simulink model "CSWI"  (Simulink 7.8)
settings: Solver=ode3  StartTime=0.0  StopTime=t_sim  FixedStep=1/6400  MaxStep=0.001  MinStep=0.000005  RelTol=1e-3
StopFcn:
  | ComtradeWrite5( RDRE1_UIabc, RDRE1_ANames, RDRE1_Dsignals, RDRE1_DNames, RDRE1_ADCscale, RDRE1_PromtFile, RDRE1_NumFile, RDRE1_FileFormat, RDRE1_TestNum);
  | clear RDRE1_UIabc RDRE1_ANames RDRE1_Dsignals RDRE1_DNames RDRE1_ADCscale  RDRE1_PromtFile RDRE1_NumFile RDRE1_FileFormat RDRE1_TestNum
values from neighbouring files (symbols this model uses):
  BlkTmms1 = 700    [CSWI_SG1.m]    (also in CSWI_SG2.m = 650; CSWI_SG3.m; CSWI_SG4.m; CSWI_SG5.m)
  BlkTmms2 = 800    [CSWI_SG1.m]    (also in CSWI_SG2.m = 750; CSWI_SG3.m; CSWI_SG4.m; CSWI_SG5.m)
  ClsTmms1 = 250    [CSWI_SG1.m]    (also in CSWI_SG2.m = 200; CSWI_SG3.m; CSWI_SG4.m; CSWI_SG5.m)
  ClsTmms2 = 170    [CSWI_SG1.m]    (also in CSWI_SG2.m = 100; CSWI_SG3.m; CSWI_SG4.m; CSWI_SG5.m)
  ClsTmms3 = 60    [CSWI_SG1.m]    (also in CSWI_SG2.m = 30; CSWI_SG3.m; CSWI_SG4.m; CSWI_SG5.m)
  ClsTmms4 = 10    [CSWI_SG1.m]    (also in CSWI_SG2.m = 20; CSWI_SG3.m; CSWI_SG4.m; CSWI_SG5.m)
  FailTmms = 350    [CSWI_SG1.m]    (also in CSWI_SG2.m = 300; CSWI_SG3.m; CSWI_SG4.m; CSWI_SG5.m)
  FctMod1 = 1    [CSWI_SG1.m]    (also in CSWI_SG2.m; CSWI_SG3.m; CSWI_SG4.m; CSWI_SG5.m)
  FctMod2 = 1    [CSWI_SG1.m]    (also in CSWI_SG2.m; CSWI_SG3.m; CSWI_SG4.m = 0; CSWI_SG5.m)
  FctMod3 = 1    [CSWI_SG1.m]    (also in CSWI_SG2.m; CSWI_SG3.m; CSWI_SG4.m; CSWI_SG5.m = 0)
  Num_SG = 1    [CSWI_generate_tests.m]
  OpnTmms1 = 300    [CSWI_SG1.m]    (also in CSWI_SG2.m = 250; CSWI_SG3.m; CSWI_SG4.m; CSWI_SG5.m)
  OpnTmms2 = 200    [CSWI_SG1.m]    (also in CSWI_SG2.m = 150; CSWI_SG3.m; CSWI_SG4.m; CSWI_SG5.m)
  OpnTmms3 = 30    [CSWI_SG1.m]    (also in CSWI_SG2.m = 90; CSWI_SG3.m = 90; CSWI_SG4.m; CSWI_SG5.m)
  test_dc = 'Ïðîâåðêà îòñóòñòâèÿ ôîðìèðîâàíèÿ ñèãíàëîâ "Âêë." ïðè ôîðìèðîâàíèè ñèãíàëà  "Îòêë. îò ÄÓ"'    [CSWI_generate_tests.m]
undefined symbols (not defined in the file or in its folder): sigbuilder_block, Test_num
libraries: powerlib_extras x21
(part 2 of 3)

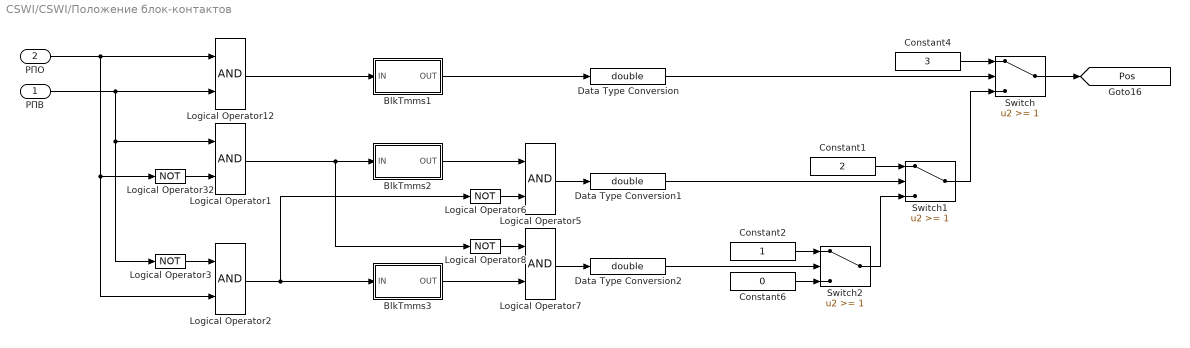
== system CSWI/CSWI/Положение блок-контактов ==
  РПВ : Inport  SampleTime=Tmega
  РПО : Inport  Port=2  SampleTime=Tmega
  BlkTmms1 : Subsystem  DialogController=POWERSYS.PowerSysDialog  mask(Discrete On/Off Delay ){type_delay=On delay, delay=0.5, ic=0, Ts=Tmega}
      mask prompts: type_delay "Type:"; delay "Time delay:"; ic "Input at t = -Ts (0/1):"; Ts "Sample time Ts:"
      mask help:
      | Apply a delay on the input signal when the input changes to TRUE (1) or FALSE (0).
      |
      | On delay: When the input becomes TRUE, the output becomes TRUE after the specified time delay as long as the input is still TRUE. If the input becomes FALSE before the time delay has expired , the output stays FALSE.
      |
      | Off delay: When the input becomes FALSE, the output becomes FALSE after the specified time delay as long as the input is still FALSE. If the input becomes TRUE before the time delay has expired , the output stays TRUE.
      |
      | The input value (0/1) at time step preceding t=0 is specified by the parameter "input at t = -Ts".
      mask init:
      | str=sprintf('%g %c',delay,'s');
      | power_initmask();
      mask Help: This block is part of a subset of blocks in the Extras library that does not have documentation associated with it, other than the block mask description.
      mask StyleString: popup(On delay|Off delay),edit,edit,edit
      mask Display:
      | plot(0,0,100,100,[10,10,10,90,90,90],[60,40,50,50,40,60]);
      | text(25+(type_delay-1)*50,80,'t');
      | text(15,20,str);
  BlkTmms2 : Subsystem  DialogController=POWERSYS.PowerSysDialog  mask(Discrete On/Off Delay ){type_delay=Off delay, delay=0.5, ic=0, Ts=Tmega}
      mask prompts: type_delay "Type:"; delay "Time delay:"; ic "Input at t = -Ts (0/1):"; Ts "Sample time Ts:"
      mask help:
      | Apply a delay on the input signal when the input changes to TRUE (1) or FALSE (0).
      |
      | On delay: When the input becomes TRUE, the output becomes TRUE after the specified time delay as long as the input is still TRUE. If the input becomes FALSE before the time delay has expired , the output stays FALSE.
      |
      | Off delay: When the input becomes FALSE, the output becomes FALSE after the specified time delay as long as the input is still FALSE. If the input becomes TRUE before the time delay has expired , the output stays TRUE.
      |
      | The input value (0/1) at time step preceding t=0 is specified by the parameter "input at t = -Ts".
      mask init:
      | str=sprintf('%g %c',delay,'s');
      | power_initmask();
      mask Help: This block is part of a subset of blocks in the Extras library that does not have documentation associated with it, other than the block mask description.
      mask StyleString: popup(On delay|Off delay),edit,edit,edit
      mask Display:
      | plot(0,0,100,100,[10,10,10,90,90,90],[60,40,50,50,40,60]);
      | text(25+(type_delay-1)*50,80,'t');
      | text(15,20,str);
  BlkTmms3 : Subsystem  DialogController=POWERSYS.PowerSysDialog  mask(Discrete On/Off Delay ){type_delay=Off delay, delay=0.5, ic=0, Ts=Tmega}
      mask prompts: type_delay "Type:"; delay "Time delay:"; ic "Input at t = -Ts (0/1):"; Ts "Sample time Ts:"
      mask help:
      | Apply a delay on the input signal when the input changes to TRUE (1) or FALSE (0).
      |
      | On delay: When the input becomes TRUE, the output becomes TRUE after the specified time delay as long as the input is still TRUE. If the input becomes FALSE before the time delay has expired , the output stays FALSE.
      |
      | Off delay: When the input becomes FALSE, the output becomes FALSE after the specified time delay as long as the input is still FALSE. If the input becomes TRUE before the time delay has expired , the output stays TRUE.
      |
      | The input value (0/1) at time step preceding t=0 is specified by the parameter "input at t = -Ts".
      mask init:
      | str=sprintf('%g %c',delay,'s');
      | power_initmask();
      mask Help: This block is part of a subset of blocks in the Extras library that does not have documentation associated with it, other than the block mask description.
      mask StyleString: popup(On delay|Off delay),edit,edit,edit
      mask Display:
      | plot(0,0,100,100,[10,10,10,90,90,90],[60,40,50,50,40,60]);
      | text(25+(type_delay-1)*50,80,'t');
      | text(15,20,str);
  Constant1 : Constant  Value=2  SampleTime=Tmega
  Constant2 : Constant  SampleTime=Tmega
  Constant4 : Constant  Value=3  SampleTime=Tmega
  Constant6 : Constant  Value=0  SampleTime=Tmega
  Data Type Conversion : DataTypeConversion  OutDataTypeStr=double  SampleTime=Tmega
  Data Type Conversion1 : DataTypeConversion  OutDataTypeStr=double  SampleTime=Tmega
  Data Type Conversion2 : DataTypeConversion  OutDataTypeStr=double  SampleTime=Tmega
  Logical Operator{1..2,5,7,12} (5 alike) : Logic  AllPortsSameDT=off  OutDataTypeStr=boolean  SampleTime=Tmega
  Logical Operator{3,6,8,32} (4 alike) : Logic  Operator=NOT  AllPortsSameDT=off  OutDataTypeStr=boolean  SampleTime=Tmega
  Switch : Switch  Threshold=1  SampleTime=Tmega
  Switch1 : Switch  Threshold=1  SampleTime=Tmega
  Switch2 : Switch  Threshold=1  SampleTime=Tmega
  tag scope: Pos=global
  wires:
  РПО/1 -> Logical Operator12/1, Logical Operator2/2, Logical Operator32/1
  РПВ/1 -> Logical Operator12/2, Logical Operator3/1, Logical Operator1/1
  Logical Operator12/1 -> BlkTmms1/1(IN)
  Logical Operator32/1 -> Logical Operator1/2
  Logical Operator3/1 -> Logical Operator2/1
  Logical Operator1/1 -> BlkTmms2/1(IN), Logical Operator8/1
  Logical Operator2/1 -> BlkTmms3/1(IN), Logical Operator6/1
  BlkTmms2/1(OUT) -> Logical Operator5/1
  Logical Operator6/1 -> Logical Operator5/2
  BlkTmms3/1(OUT) -> Logical Operator7/2
  Logical Operator8/1 -> Logical Operator7/1
  BlkTmms1/1(OUT) -> Data Type Conversion/1
  Constant4/1 -> Switch/1
  Constant1/1 -> Switch1/1
  Logical Operator5/1 -> Data Type Conversion1/1
  Switch1/1 -> Switch/3
  Data Type Conversion/1 -> Switch/2
  Data Type Conversion1/1 -> Switch1/2
  Switch2/1 -> Switch1/3
  Logical Operator7/1 -> Data Type Conversion2/1
  Data Type Conversion2/1 -> Switch2/2
  Constant2/1 -> Switch2/1
  Switch/1 -> [Pos]
  Constant6/1 -> Switch2/3

== system CSWI/CSWI/РФК и Аварийное отключение ==
  Вывод ОУ : Inport  SampleTime=Tmega
  РПВ : Inport  Port=2  SampleTime=Tmega
  РПО : Inport  Port=3  SampleTime=Tmega
  Опер. Откл. : Inport  Port=4  SampleTime=Tmega
  Discrete Bistable7 : Subsystem  DialogController=POWERSYS.PowerSysDialog  mask(Discrete Bistable Flip-Flop (Priority to Set or Reset)){SPSpriority=Reset, ic=0, Ts=Tmega}
      mask prompts: SPSpriority "Priority to input:"; ic "Initial Q output (0/1):"; Ts "Sample time:"
      mask help:
      | SR Flip-Flop block, with priority given either  to the Set  (S) or Reset  (R) input.
      |
      | Priority to Set: If inputs S (set) and R (reset) are TRUE (1) simultaneously, the output Q is set to TRUE (1).
      |
      | Priority to Reset: If inputs S (set) and R (reset) are TRUE (1) simultaneously, the output Q is reset to FALSE (0).
      |
      | The  Q! output  is the complement of the Q output.
      | The initial value of the Q output  is specified by the parameter "Initial Q output".
      mask init:
      | if (SPSpriority==1)   % RESET
      |  str1 = '[R]';
      |  str2 = 'S';
      | else
      | str1= 'R';
      | str2 = '[S]';
      | end
      | power_initmask();
      mask Help: This block is part of a subset of blocks in the Extras library that does not have documentation associated with it, other than the block mask description.
      mask StyleString: popup(Reset|Set),edit,edit
      mask Display:
      | plot(0,0,100,100);
      | text(8,25,str1);
      | text(8,75,str2);
      | text(72,50,'Q');
  Logical Operator29 : Logic  Operator=OR  AllPortsSameDT=off  OutDataTypeStr=boolean  SampleTime=Tmega
  Logical Operator39 : Logic  AllPortsSameDT=off  OutDataTypeStr=boolean  SampleTime=Tmega
  Logical Operator40 : Logic  AllPortsSameDT=off  OutDataTypeStr=boolean  SampleTime=Tmega
  T. Авар. откл. : powerlib_extras/Discrete  Control Blocks/Discrete On//Off Delay  type_delay=On delay  delay=FailTmms  ic=0  Ts=Tmega
  РФК : Outport  SampleTime=Tmega
  Авар. откл. : Outport  Port=2  SampleTime=Tmega
  wires:
  Logical Operator29/1 -> Discrete Bistable7/2(R)
  РПО/1 -> Logical Operator39/2, Logical Operator40/2
  Discrete Bistable7/1(Q) -> Logical Operator40/1, РФК/1
  Logical Operator40/1 -> T. Авар. откл./1
  Вывод ОУ/1 -> Logical Operator39/1
  РПВ/1 -> Discrete Bistable7/1(S)
  T. Авар. откл./1 -> Авар. откл./1
  Logical Operator39/1 -> Logical Operator29/2
  Опер. Откл./1 -> Logical Operator29/1

== system CSWI/DREGOUT1/Signal Builder ==
  Demux : Demux  Tag=STV Demux  Outputs=1
  FromWs : FromWorkspace  Tag=STV FromWs  VariableName=tuvar  SampleTime=0  SigBuilderData=DataTag0  VnvData=DataTag1
      SigBuilderData=|
      | common.afterFinalStr = 'Extrapolate'
      | common.sampleTime = 0
      | dataSet.timeRange = [0 5]
      | dataSet.name = 'Group 1'
      | sbobj.Groups.Name = 'Group 1'
      | sbobj.Groups.Signals.Name = 'Pusk Osc'
      | sbobj.Groups.Signals.XData = [0 0.5 0.5 0.54 0.54 5]
      | sbobj.Groups.Signals.YData = [0 0 1 1 0 0]
      | sbobj.Groups.TimeRange = [0 5]
  Pusk Osc : Outport  Tag=STV Outport
  wires:
  FromWs/1 -> Demux/1
  Demux/1 -> Pusk Osc/1

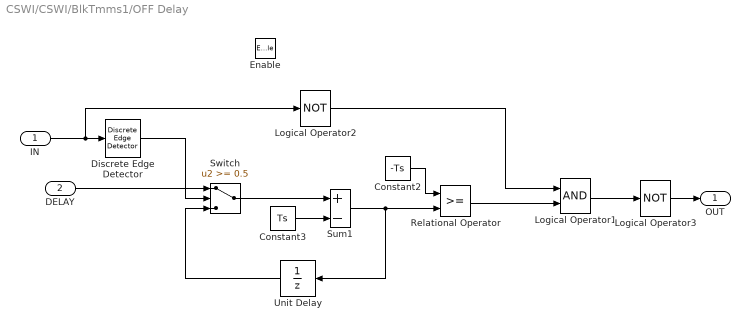
== system CSWI/CSWI/BlkTmms1/OFF Delay ==
  IN : Inport
  DELAY : Inport  Port=2
  Enable : EnablePort  PropagateVarSize=During execution
  Constant2 : Constant  Value=-Ts
  Constant3 : Constant  Value=Ts
  Discrete Edge Detector : powerlib_extras/Discrete  Control Blocks/Discrete Edge Detector  model=Falling  ic=ic  Ts=Ts
  Logical Operator1 : Logic
  Logical Operator2 : Logic  Operator=NOT
  Logical Operator3 : Logic  Operator=NOT
  Relational Operator : RelationalOperator  OutDataTypeStr=boolean  InputSameDT=on
  Sum1 : Sum  Inputs=+-  SaturateOnIntegerOverflow=on  InputSameDT=on  OutDataTypeStr=Inherit: Same as first input
  Switch : Switch  Threshold=0.5  SaturateOnIntegerOverflow=on  InputSameDT=on
  Unit Delay : UnitDelay  SampleTime=Ts
  OUT : Outport
  wires:
  Unit Delay/1 -> Switch/3
  Sum1/1 -> Relational Operator/2, Unit Delay/1
  Switch/1 -> Sum1/1
  Constant3/1 -> Sum1/2
  Relational Operator/1 -> Logical Operator1/2
  IN/1 -> Discrete Edge Detector/1, Logical Operator2/1
  Logical Operator1/1 -> Logical Operator3/1
  DELAY/1 -> Switch/1
  Discrete Edge Detector/1 -> Switch/2
  Constant2/1 -> Relational Operator/1
  Logical Operator2/1 -> Logical Operator1/1
  Logical Operator3/1 -> OUT/1

== system CSWI/CSWI/BlkTmms1/ON Delay ==
  IN : Inport
  DELAY : Inport  Port=2
  Enable : EnablePort  PropagateVarSize=During execution
  Constant2 : Constant  Value=-Ts
  Constant3 : Constant  Value=Ts
  Discrete Edge Detector : powerlib_extras/Discrete  Control Blocks/Discrete Edge Detector  model=Rising  ic=ic  Ts=Ts
  Logical Operator1 : Logic
  Relational Operator : RelationalOperator  OutDataTypeStr=boolean  InputSameDT=on
  Sum1 : Sum  Inputs=+-  SaturateOnIntegerOverflow=on  InputSameDT=on  OutDataTypeStr=Inherit: Same as first input
  Switch : Switch  Threshold=0.5  SaturateOnIntegerOverflow=on  InputSameDT=on
  Unit Delay : UnitDelay  SampleTime=Ts
  OUT : Outport
  wires:
  Unit Delay/1 -> Switch/3
  Sum1/1 -> Unit Delay/1, Relational Operator/2
  Switch/1 -> Sum1/1
  Constant3/1 -> Sum1/2
  Relational Operator/1 -> Logical Operator1/2
  IN/1 -> Discrete Edge Detector/1, Logical Operator1/1
  Logical Operator1/1 -> OUT/1
  DELAY/1 -> Switch/1
  Discrete Edge Detector/1 -> Switch/2
  Constant2/1 -> Relational Operator/1

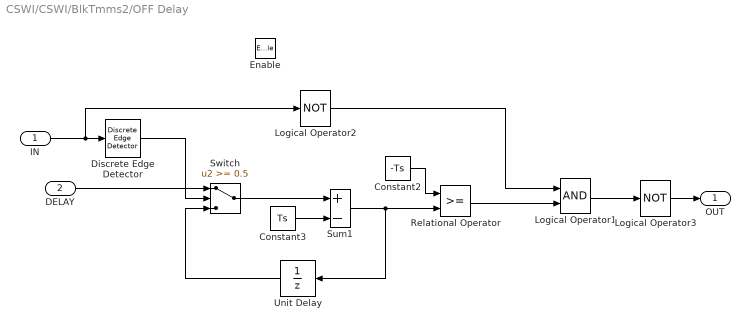
== system CSWI/CSWI/BlkTmms2/OFF Delay ==
  IN : Inport
  DELAY : Inport  Port=2
  Enable : EnablePort  PropagateVarSize=During execution
  Constant2 : Constant  Value=-Ts
  Constant3 : Constant  Value=Ts
  Discrete Edge Detector : powerlib_extras/Discrete  Control Blocks/Discrete Edge Detector  model=Falling  ic=ic  Ts=Ts
  Logical Operator1 : Logic
  Logical Operator2 : Logic  Operator=NOT
  Logical Operator3 : Logic  Operator=NOT
  Relational Operator : RelationalOperator  OutDataTypeStr=boolean  InputSameDT=on
  Sum1 : Sum  Inputs=+-  SaturateOnIntegerOverflow=on  InputSameDT=on  OutDataTypeStr=Inherit: Same as first input
  Switch : Switch  Threshold=0.5  SaturateOnIntegerOverflow=on  InputSameDT=on
  Unit Delay : UnitDelay  SampleTime=Ts
  OUT : Outport
  wires:
  Unit Delay/1 -> Switch/3
  Sum1/1 -> Relational Operator/2, Unit Delay/1
  Switch/1 -> Sum1/1
  Constant3/1 -> Sum1/2
  Relational Operator/1 -> Logical Operator1/2
  IN/1 -> Discrete Edge Detector/1, Logical Operator2/1
  Logical Operator1/1 -> Logical Operator3/1
  DELAY/1 -> Switch/1
  Discrete Edge Detector/1 -> Switch/2
  Constant2/1 -> Relational Operator/1
  Logical Operator2/1 -> Logical Operator1/1
  Logical Operator3/1 -> OUT/1

== system CSWI/CSWI/BlkTmms2/ON Delay ==
  IN : Inport
  DELAY : Inport  Port=2
  Enable : EnablePort  PropagateVarSize=During execution
  Constant2 : Constant  Value=-Ts
  Constant3 : Constant  Value=Ts
  Discrete Edge Detector : powerlib_extras/Discrete  Control Blocks/Discrete Edge Detector  model=Rising  ic=ic  Ts=Ts
  Logical Operator1 : Logic
  Relational Operator : RelationalOperator  OutDataTypeStr=boolean  InputSameDT=on
  Sum1 : Sum  Inputs=+-  SaturateOnIntegerOverflow=on  InputSameDT=on  OutDataTypeStr=Inherit: Same as first input
  Switch : Switch  Threshold=0.5  SaturateOnIntegerOverflow=on  InputSameDT=on
  Unit Delay : UnitDelay  SampleTime=Ts
  OUT : Outport
  wires:
  Unit Delay/1 -> Switch/3
  Sum1/1 -> Unit Delay/1, Relational Operator/2
  Switch/1 -> Sum1/1
  Constant3/1 -> Sum1/2
  Relational Operator/1 -> Logical Operator1/2
  IN/1 -> Discrete Edge Detector/1, Logical Operator1/1
  Logical Operator1/1 -> OUT/1
  DELAY/1 -> Switch/1
  Discrete Edge Detector/1 -> Switch/2
  Constant2/1 -> Relational Operator/1

== system CSWI/CSWI/Блок включения/ClsTmms1 ==
  note: Silvano Casoria
      | Power System Simulation Laboratory
      | IREQ, Hydro-Quebc
  note: Discrete On/Off Delay
  IN : Inport
  Constant : Constant
  Constant1 : Constant  Value=delay - eps
  Constant2 : Constant  Value=type_delay
  Data Type Conversion1 : DataTypeConversion  OutDataTypeStr=boolean  SaturateOnIntegerOverflow=on  RndMeth=Zero
  Logical Operator1 : Logic  Operator=OR
  Logical Operator2 : Logic  Operator=NOT  Inputs=1
  OFF Delay : Subsystem  TreatAsAtomicUnit=on
  ON Delay : Subsystem  TreatAsAtomicUnit=on
  Relational Operator1 : RelationalOperator  Operator===  InputSameDT=on
  OUT : Outport
  wires:
  Data Type Conversion1/1 -> ON Delay/1(IN), OFF Delay/1(IN)
  Constant/1 -> Relational Operator1/2
  Relational Operator1/1 -> ON Delay/Enable, Logical Operator2/1
  Constant2/1 -> Relational Operator1/1
  Logical Operator2/1 -> OFF Delay/Enable
  OFF Delay/1(OUT) -> Logical Operator1/2
  ON Delay/1(OUT) -> Logical Operator1/1
  Logical Operator1/1 -> OUT/1
  Constant1/1 -> ON Delay/2(DELAY), OFF Delay/2(DELAY)
  IN/1 -> Data Type Conversion1/1

== system CSWI/CSWI/Блок включения/ClsTmms2 ==
  note: Discrete Monostable
  note: Silvano Casoria
      | Power System Simulation Laboratory
      | IREQ, Hydro-Quebc
  In : Inport
  Constant2 : Constant  Value=-Ts
  Constant3 : Constant  Value=Ts
  Edge_Detector : Subsystem  mask(Discrete Edge Detector){model=EdgeDetect, ic=ic, Ts=Ts}
      mask prompts: model "Edge:"; ic "Input at t = -Ts:"; Ts "Sample time Ts:"
      mask help:
      | This block compares its present input to its previous input.
      |
      | If the input  is a logic signal (TRUE (1) or FALSE (0), the output is a one-step boolean signal TRUE  when  the specified edge (Rising, Falling or Either)  is detected.
      |
      | This block can also be used to detect the slope polarity of a continuous signal. For example, if the specified edge is  "Rising", the output is TRUE as long as the slope of the input signal is positive.
      |
      | The input value at time step preceding t=0 is specified by the parameter "Input at t=-Ts"
      mask init:
      | if model~=3,
      | 	x1 = (model -1)*20;
      |     x2 = (model -1)*60;
      | 	X1=[5,20,20,35]+25; Y1=[20+x2,20+x2,80-x2,80-x2];
      | 	X2=[5,20,35]+25;    Y2=[40+x1,60-x1,40+x1];
      | 	X3=[];X4=[];Y3=[];Y4=[];
      | else
      | 	x1 = 20;
      | 	x2 = 60;
      | 	X1=[5,20,20,35]+8; Y1=[20,20,80,80];
      | 	X2=[5,20,35]+8;    Y2=[40,60,40];
      | 	X3=[5,20,20,35]+53; Y3=[20+x2,20+x2,80-x2,80-x2];
      | 	X4=[5,20,35]+53;    Y4=[40+x1,60-x1,40+x1];
      | end
      mask Display: plot(0,0,100,100, X1,Y1,X2,Y2,X3,Y3,X4,Y4);
  Logical Operator1 : Logic
  Logical Operator2 : Logic  Operator=NOT  Inputs=1
  Relational Operator : RelationalOperator  Operator=>  InputSameDT=on
  Sum1 : Sum  Inputs=+-  SaturateOnIntegerOverflow=on  InputSameDT=on  OutDataTypeStr=Inherit: Same as first input
  Switch : Switch  Threshold=0.5  SaturateOnIntegerOverflow=on  InputSameDT=on
  T_monostable : Constant  Value=t_mono-eps
  Unit Delay : UnitDelay  SampleTime=Ts
  delay : UnitDelay  SampleTime=Ts
  Out : Outport
  wires:
  Sum1/1 -> Unit Delay/1, Relational Operator/1
  Unit Delay/1 -> Switch/3
  Constant3/1 -> Sum1/2
  Switch/1 -> Sum1/1
  T_monostable/1 -> Switch/1
  In/1 -> Edge_Detector/1(In)
  Relational Operator/1 -> delay/1, Out/1
  Logical Operator1/1 -> Switch/2
  delay/1 -> Logical Operator2/1
  Logical Operator2/1 -> Logical Operator1/1
  Edge_Detector/1(Out) -> Logical Operator1/2
  Constant2/1 -> Relational Operator/2

== system CSWI/CSWI/Блок включения/ClsTmms3 ==
  note: Silvano Casoria
      | Power System Simulation Laboratory
      | IREQ, Hydro-Quebc
  note: Discrete On/Off Delay
  IN : Inport
  Constant : Constant
  Constant1 : Constant  Value=delay - eps
  Constant2 : Constant  Value=type_delay
  Data Type Conversion1 : DataTypeConversion  OutDataTypeStr=boolean  SaturateOnIntegerOverflow=on  RndMeth=Zero
  Logical Operator1 : Logic  Operator=OR
  Logical Operator2 : Logic  Operator=NOT  Inputs=1
  OFF Delay : Subsystem  TreatAsAtomicUnit=on
  ON Delay : Subsystem  TreatAsAtomicUnit=on
  Relational Operator1 : RelationalOperator  Operator===  InputSameDT=on
  OUT : Outport
  wires:
  Data Type Conversion1/1 -> ON Delay/1(IN), OFF Delay/1(IN)
  Constant/1 -> Relational Operator1/2
  Relational Operator1/1 -> ON Delay/Enable, Logical Operator2/1
  Constant2/1 -> Relational Operator1/1
  Logical Operator2/1 -> OFF Delay/Enable
  OFF Delay/1(OUT) -> Logical Operator1/2
  ON Delay/1(OUT) -> Logical Operator1/1
  Logical Operator1/1 -> OUT/1
  Constant1/1 -> ON Delay/2(DELAY), OFF Delay/2(DELAY)
  IN/1 -> Data Type Conversion1/1

== system CSWI/CSWI/Блок включения/ClsTmms4 ==
  note: Silvano Casoria
      | Power System Simulation Laboratory
      | IREQ, Hydro-Quebc
  note: Discrete On/Off Delay
  IN : Inport
  Constant : Constant
  Constant1 : Constant  Value=delay - eps
  Constant2 : Constant  Value=type_delay
  Data Type Conversion1 : DataTypeConversion  OutDataTypeStr=boolean  SaturateOnIntegerOverflow=on  RndMeth=Zero
  Logical Operator1 : Logic  Operator=OR
  Logical Operator2 : Logic  Operator=NOT  Inputs=1
  OFF Delay : Subsystem  TreatAsAtomicUnit=on
  ON Delay : Subsystem  TreatAsAtomicUnit=on
  Relational Operator1 : RelationalOperator  Operator===  InputSameDT=on
  OUT : Outport
  wires:
  Data Type Conversion1/1 -> ON Delay/1(IN), OFF Delay/1(IN)
  Constant/1 -> Relational Operator1/2
  Relational Operator1/1 -> ON Delay/Enable, Logical Operator2/1
  Constant2/1 -> Relational Operator1/1
  Logical Operator2/1 -> OFF Delay/Enable
  OFF Delay/1(OUT) -> Logical Operator1/2
  ON Delay/1(OUT) -> Logical Operator1/1
  Logical Operator1/1 -> OUT/1
  Constant1/1 -> ON Delay/2(DELAY), OFF Delay/2(DELAY)
  IN/1 -> Data Type Conversion1/1

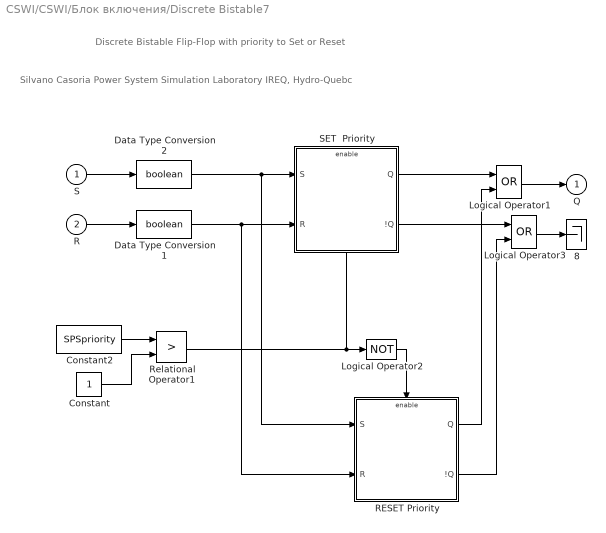
== system CSWI/CSWI/Блок включения/Discrete Bistable7 ==
  note: Silvano Casoria
      | Power System Simulation Laboratory
      | IREQ, Hydro-Quebc
  note: Discrete Bistable Flip-Flop with priority to Set or Reset
  S : Inport
  R : Inport  Port=2
  8 : Terminator
  Constant : Constant
  Constant2 : Constant  Value=SPSpriority
  Data Type Conversion1 : DataTypeConversion  OutDataTypeStr=boolean  SaturateOnIntegerOverflow=on  RndMeth=Zero
  Data Type Conversion2 : DataTypeConversion  OutDataTypeStr=boolean  SaturateOnIntegerOverflow=on  RndMeth=Zero
  Logical Operator1 : Logic  Operator=OR
  Logical Operator2 : Logic  Operator=NOT  Inputs=1
  Logical Operator3 : Logic  Operator=OR
  RESET Priority : Subsystem  TreatAsAtomicUnit=on
  Relational Operator1 : RelationalOperator  Operator=>  InputSameDT=on
  SET  Priority : Subsystem  TreatAsAtomicUnit=on
  Q : Outport  InitialOutput=0
  wires:
  RESET Priority/2(!Q) -> Logical Operator3/2
  RESET Priority/1(Q) -> Logical Operator1/2
  Logical Operator3/1 -> 8/1
  SET  Priority/2(!Q) -> Logical Operator3/1
  Logical Operator1/1 -> Q/1
  SET  Priority/1(Q) -> Logical Operator1/1
  Constant/1 -> Relational Operator1/2
  Relational Operator1/1 -> SET  Priority/Enable, Logical Operator2/1
  Constant2/1 -> Relational Operator1/1
  Logical Operator2/1 -> RESET Priority/Enable
  Data Type Conversion1/1 -> SET  Priority/2(R), RESET Priority/2(R)
  Data Type Conversion2/1 -> SET  Priority/1(S), RESET Priority/1(S)
  S/1 -> Data Type Conversion2/1
  R/1 -> Data Type Conversion1/1

== system CSWI/CSWI/Блок отключения/OpnTmms1 ==
  note: Silvano Casoria
      | Power System Simulation Laboratory
      | IREQ, Hydro-Quebc
  note: Discrete On/Off Delay
  IN : Inport
  Constant : Constant
  Constant1 : Constant  Value=delay - eps
  Constant2 : Constant  Value=type_delay
  Data Type Conversion1 : DataTypeConversion  OutDataTypeStr=boolean  SaturateOnIntegerOverflow=on  RndMeth=Zero
  Logical Operator1 : Logic  Operator=OR
  Logical Operator2 : Logic  Operator=NOT  Inputs=1
  OFF Delay : Subsystem  TreatAsAtomicUnit=on
  ON Delay : Subsystem  TreatAsAtomicUnit=on
  Relational Operator1 : RelationalOperator  Operator===  InputSameDT=on
  OUT : Outport
  wires:
  Data Type Conversion1/1 -> ON Delay/1(IN), OFF Delay/1(IN)
  Constant/1 -> Relational Operator1/2
  Relational Operator1/1 -> ON Delay/Enable, Logical Operator2/1
  Constant2/1 -> Relational Operator1/1
  Logical Operator2/1 -> OFF Delay/Enable
  OFF Delay/1(OUT) -> Logical Operator1/2
  ON Delay/1(OUT) -> Logical Operator1/1
  Logical Operator1/1 -> OUT/1
  Constant1/1 -> ON Delay/2(DELAY), OFF Delay/2(DELAY)
  IN/1 -> Data Type Conversion1/1

== system CSWI/CSWI/Блок отключения/OpnTmms2 ==
  note: Discrete Monostable
  note: Silvano Casoria
      | Power System Simulation Laboratory
      | IREQ, Hydro-Quebc
  In : Inport
  Constant2 : Constant  Value=-Ts
  Constant3 : Constant  Value=Ts
  Edge_Detector : Subsystem  mask(Discrete Edge Detector){model=EdgeDetect, ic=ic, Ts=Ts}
      mask prompts: model "Edge:"; ic "Input at t = -Ts:"; Ts "Sample time Ts:"
      mask help:
      | This block compares its present input to its previous input.
      |
      | If the input  is a logic signal (TRUE (1) or FALSE (0), the output is a one-step boolean signal TRUE  when  the specified edge (Rising, Falling or Either)  is detected.
      |
      | This block can also be used to detect the slope polarity of a continuous signal. For example, if the specified edge is  "Rising", the output is TRUE as long as the slope of the input signal is positive.
      |
      | The input value at time step preceding t=0 is specified by the parameter "Input at t=-Ts"
      mask init: same as CSWI/CSWI/Блок включения/ClsTmms2/Edge_Detector
      mask Display: plot(0,0,100,100, X1,Y1,X2,Y2,X3,Y3,X4,Y4);
  Logical Operator1 : Logic
  Logical Operator2 : Logic  Operator=NOT  Inputs=1
  Relational Operator : RelationalOperator  Operator=>  InputSameDT=on
  Sum1 : Sum  Inputs=+-  SaturateOnIntegerOverflow=on  InputSameDT=on  OutDataTypeStr=Inherit: Same as first input
  Switch : Switch  Threshold=0.5  SaturateOnIntegerOverflow=on  InputSameDT=on
  T_monostable : Constant  Value=t_mono-eps
  Unit Delay : UnitDelay  SampleTime=Ts
  delay : UnitDelay  SampleTime=Ts
  Out : Outport
  wires:
  Sum1/1 -> Unit Delay/1, Relational Operator/1
  Unit Delay/1 -> Switch/3
  Constant3/1 -> Sum1/2
  Switch/1 -> Sum1/1
  T_monostable/1 -> Switch/1
  In/1 -> Edge_Detector/1(In)
  Relational Operator/1 -> delay/1, Out/1
  Logical Operator1/1 -> Switch/2
  delay/1 -> Logical Operator2/1
  Logical Operator2/1 -> Logical Operator1/1
  Edge_Detector/1(Out) -> Logical Operator1/2
  Constant2/1 -> Relational Operator/2

== system CSWI/CSWI/Блок отключения/OpnTmms3 ==
  note: Silvano Casoria
      | Power System Simulation Laboratory
      | IREQ, Hydro-Quebc
  note: Discrete On/Off Delay
  IN : Inport
  Constant : Constant
  Constant1 : Constant  Value=delay - eps
  Constant2 : Constant  Value=type_delay
  Data Type Conversion1 : DataTypeConversion  OutDataTypeStr=boolean  SaturateOnIntegerOverflow=on  RndMeth=Zero
  Logical Operator1 : Logic  Operator=OR
  Logical Operator2 : Logic  Operator=NOT  Inputs=1
  OFF Delay : Subsystem  TreatAsAtomicUnit=on
  ON Delay : Subsystem  TreatAsAtomicUnit=on
  Relational Operator1 : RelationalOperator  Operator===  InputSameDT=on
  OUT : Outport
  wires:
  Data Type Conversion1/1 -> ON Delay/1(IN), OFF Delay/1(IN)
  Constant/1 -> Relational Operator1/2
  Relational Operator1/1 -> ON Delay/Enable, Logical Operator2/1
  Constant2/1 -> Relational Operator1/1
  Logical Operator2/1 -> OFF Delay/Enable
  OFF Delay/1(OUT) -> Logical Operator1/2
  ON Delay/1(OUT) -> Logical Operator1/1
  Logical Operator1/1 -> OUT/1
  Constant1/1 -> ON Delay/2(DELAY), OFF Delay/2(DELAY)
  IN/1 -> Data Type Conversion1/1

== system CSWI/CSWI/Положение блок-контактов/BlkTmms1 ==
  note: Silvano Casoria
      | Power System Simulation Laboratory
      | IREQ, Hydro-Quebc
  note: Discrete On/Off Delay
  IN : Inport  SampleTime=Tmega
  Constant : Constant  SampleTime=Tmega
  Constant1 : Constant  Value=delay - eps  SampleTime=Tmega
  Constant2 : Constant  Value=type_delay  SampleTime=Tmega
  Data Type Conversion1 : DataTypeConversion  OutDataTypeStr=boolean  SampleTime=Tmega  SaturateOnIntegerOverflow=on  RndMeth=Zero
  Logical Operator1 : Logic  Operator=OR  SampleTime=Tmega
  Logical Operator2 : Logic  Operator=NOT  Inputs=1  SampleTime=Tmega
  OFF Delay : Subsystem  TreatAsAtomicUnit=on
  ON Delay : Subsystem  TreatAsAtomicUnit=on
  Relational Operator1 : RelationalOperator  Operator===  SampleTime=Tmega  InputSameDT=on
  OUT : Outport  SampleTime=Tmega
  wires:
  Data Type Conversion1/1 -> ON Delay/1(IN), OFF Delay/1(IN)
  Constant/1 -> Relational Operator1/2
  Relational Operator1/1 -> ON Delay/Enable, Logical Operator2/1
  Constant2/1 -> Relational Operator1/1
  Logical Operator2/1 -> OFF Delay/Enable
  OFF Delay/1(OUT) -> Logical Operator1/2
  ON Delay/1(OUT) -> Logical Operator1/1
  Logical Operator1/1 -> OUT/1
  Constant1/1 -> ON Delay/2(DELAY), OFF Delay/2(DELAY)
  IN/1 -> Data Type Conversion1/1

== system CSWI/CSWI/Положение блок-контактов/BlkTmms2 ==
  note: Silvano Casoria
      | Power System Simulation Laboratory
      | IREQ, Hydro-Quebc
  note: Discrete On/Off Delay
  IN : Inport  SampleTime=Tmega
  Constant : Constant  SampleTime=Tmega
  Constant1 : Constant  Value=delay - eps  SampleTime=Tmega
  Constant2 : Constant  Value=type_delay  SampleTime=Tmega
  Data Type Conversion1 : DataTypeConversion  OutDataTypeStr=boolean  SampleTime=Tmega  SaturateOnIntegerOverflow=on  RndMeth=Zero
  Logical Operator1 : Logic  Operator=OR  SampleTime=Tmega
  Logical Operator2 : Logic  Operator=NOT  Inputs=1  SampleTime=Tmega
  OFF Delay : Subsystem  TreatAsAtomicUnit=on
  ON Delay : Subsystem  TreatAsAtomicUnit=on
  Relational Operator1 : RelationalOperator  Operator===  SampleTime=Tmega  InputSameDT=on
  OUT : Outport  SampleTime=Tmega
  wires:
  Data Type Conversion1/1 -> ON Delay/1(IN), OFF Delay/1(IN)
  Constant/1 -> Relational Operator1/2
  Relational Operator1/1 -> ON Delay/Enable, Logical Operator2/1
  Constant2/1 -> Relational Operator1/1
  Logical Operator2/1 -> OFF Delay/Enable
  OFF Delay/1(OUT) -> Logical Operator1/2
  ON Delay/1(OUT) -> Logical Operator1/1
  Logical Operator1/1 -> OUT/1
  Constant1/1 -> ON Delay/2(DELAY), OFF Delay/2(DELAY)
  IN/1 -> Data Type Conversion1/1

== system CSWI/CSWI/Положение блок-контактов/BlkTmms3 ==
  note: Silvano Casoria
      | Power System Simulation Laboratory
      | IREQ, Hydro-Quebc
  note: Discrete On/Off Delay
  IN : Inport  SampleTime=Tmega
  Constant : Constant  SampleTime=Tmega
  Constant1 : Constant  Value=delay - eps  SampleTime=Tmega
  Constant2 : Constant  Value=type_delay  SampleTime=Tmega
  Data Type Conversion1 : DataTypeConversion  OutDataTypeStr=boolean  SampleTime=Tmega  SaturateOnIntegerOverflow=on  RndMeth=Zero
  Logical Operator1 : Logic  Operator=OR  SampleTime=Tmega
  Logical Operator2 : Logic  Operator=NOT  Inputs=1  SampleTime=Tmega
  OFF Delay : Subsystem  TreatAsAtomicUnit=on
  ON Delay : Subsystem  TreatAsAtomicUnit=on
  Relational Operator1 : RelationalOperator  Operator===  SampleTime=Tmega  InputSameDT=on
  OUT : Outport  SampleTime=Tmega
  wires:
  Data Type Conversion1/1 -> ON Delay/1(IN), OFF Delay/1(IN)
  Constant/1 -> Relational Operator1/2
  Relational Operator1/1 -> ON Delay/Enable, Logical Operator2/1
  Constant2/1 -> Relational Operator1/1
  Logical Operator2/1 -> OFF Delay/Enable
  OFF Delay/1(OUT) -> Logical Operator1/2
  ON Delay/1(OUT) -> Logical Operator1/1
  Logical Operator1/1 -> OUT/1
  Constant1/1 -> ON Delay/2(DELAY), OFF Delay/2(DELAY)
  IN/1 -> Data Type Conversion1/1

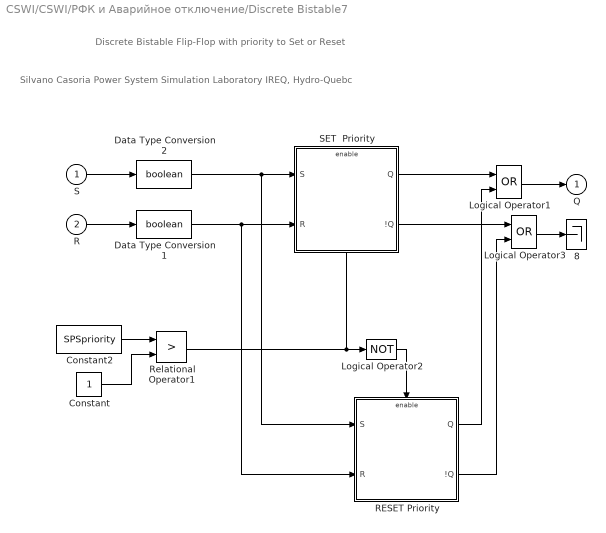
== system CSWI/CSWI/РФК и Аварийное отключение/Discrete Bistable7 ==
  note: Silvano Casoria
      | Power System Simulation Laboratory
      | IREQ, Hydro-Quebc
  note: Discrete Bistable Flip-Flop with priority to Set or Reset
  S : Inport
  R : Inport  Port=2
  8 : Terminator
  Constant : Constant
  Constant2 : Constant  Value=SPSpriority
  Data Type Conversion1 : DataTypeConversion  OutDataTypeStr=boolean  SaturateOnIntegerOverflow=on  RndMeth=Zero
  Data Type Conversion2 : DataTypeConversion  OutDataTypeStr=boolean  SaturateOnIntegerOverflow=on  RndMeth=Zero
  Logical Operator1 : Logic  Operator=OR
  Logical Operator2 : Logic  Operator=NOT  Inputs=1
  Logical Operator3 : Logic  Operator=OR
  RESET Priority : Subsystem  TreatAsAtomicUnit=on
  Relational Operator1 : RelationalOperator  Operator=>  InputSameDT=on
  SET  Priority : Subsystem  TreatAsAtomicUnit=on
  Q : Outport  InitialOutput=0
  wires:
  RESET Priority/2(!Q) -> Logical Operator3/2
  RESET Priority/1(Q) -> Logical Operator1/2
  Logical Operator3/1 -> 8/1
  SET  Priority/2(!Q) -> Logical Operator3/1
  Logical Operator1/1 -> Q/1
  SET  Priority/1(Q) -> Logical Operator1/1
  Constant/1 -> Relational Operator1/2
  Relational Operator1/1 -> SET  Priority/Enable, Logical Operator2/1
  Constant2/1 -> Relational Operator1/1
  Logical Operator2/1 -> RESET Priority/Enable
  Data Type Conversion1/1 -> SET  Priority/2(R), RESET Priority/2(R)
  Data Type Conversion2/1 -> SET  Priority/1(S), RESET Priority/1(S)
  S/1 -> Data Type Conversion2/1
  R/1 -> Data Type Conversion1/1

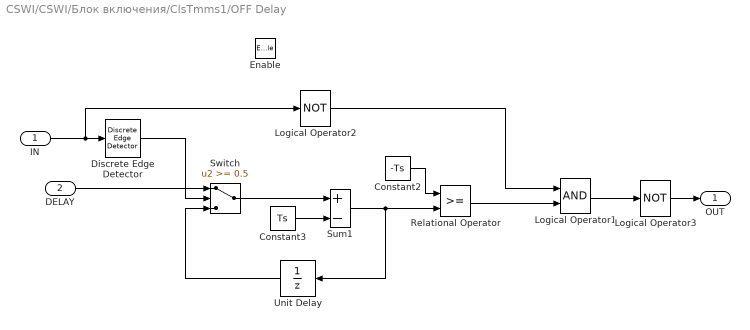
== system CSWI/CSWI/Блок включения/ClsTmms1/OFF Delay ==
  IN : Inport
  DELAY : Inport  Port=2
  Enable : EnablePort  PropagateVarSize=During execution
  Constant2 : Constant  Value=-Ts
  Constant3 : Constant  Value=Ts
  Discrete Edge Detector : powerlib_extras/Discrete  Control Blocks/Discrete Edge Detector  model=Falling  ic=ic  Ts=Ts
  Logical Operator1 : Logic
  Logical Operator2 : Logic  Operator=NOT
  Logical Operator3 : Logic  Operator=NOT
  Relational Operator : RelationalOperator  OutDataTypeStr=boolean  InputSameDT=on
  Sum1 : Sum  Inputs=+-  SaturateOnIntegerOverflow=on  InputSameDT=on  OutDataTypeStr=Inherit: Same as first input
  Switch : Switch  Threshold=0.5  SaturateOnIntegerOverflow=on  InputSameDT=on
  Unit Delay : UnitDelay  SampleTime=Ts
  OUT : Outport
  wires:
  Unit Delay/1 -> Switch/3
  Sum1/1 -> Relational Operator/2, Unit Delay/1
  Switch/1 -> Sum1/1
  Constant3/1 -> Sum1/2
  Relational Operator/1 -> Logical Operator1/2
  IN/1 -> Discrete Edge Detector/1, Logical Operator2/1
  Logical Operator1/1 -> Logical Operator3/1
  DELAY/1 -> Switch/1
  Discrete Edge Detector/1 -> Switch/2
  Constant2/1 -> Relational Operator/1
  Logical Operator2/1 -> Logical Operator1/1
  Logical Operator3/1 -> OUT/1

== system CSWI/CSWI/Блок включения/ClsTmms1/ON Delay ==
  IN : Inport
  DELAY : Inport  Port=2
  Enable : EnablePort  PropagateVarSize=During execution
  Constant2 : Constant  Value=-Ts
  Constant3 : Constant  Value=Ts
  Discrete Edge Detector : powerlib_extras/Discrete  Control Blocks/Discrete Edge Detector  model=Rising  ic=ic  Ts=Ts
  Logical Operator1 : Logic
  Relational Operator : RelationalOperator  OutDataTypeStr=boolean  InputSameDT=on
  Sum1 : Sum  Inputs=+-  SaturateOnIntegerOverflow=on  InputSameDT=on  OutDataTypeStr=Inherit: Same as first input
  Switch : Switch  Threshold=0.5  SaturateOnIntegerOverflow=on  InputSameDT=on
  Unit Delay : UnitDelay  SampleTime=Ts
  OUT : Outport
  wires:
  Unit Delay/1 -> Switch/3
  Sum1/1 -> Unit Delay/1, Relational Operator/2
  Switch/1 -> Sum1/1
  Constant3/1 -> Sum1/2
  Relational Operator/1 -> Logical Operator1/2
  IN/1 -> Discrete Edge Detector/1, Logical Operator1/1
  Logical Operator1/1 -> OUT/1
  DELAY/1 -> Switch/1
  Discrete Edge Detector/1 -> Switch/2
  Constant2/1 -> Relational Operator/1

== system CSWI/CSWI/Блок включения/ClsTmms2/Edge_Detector ==
  note: Edge or Slope Detector
  note: Silvano Casoria
      | Power System Simulation Laboratory
      | IREQ, Hydro-Quebc
  In : Inport
  Constant1 : Constant  Value=model
  Demux : Demux  Outputs=2
  Logical Operator1 : Logic  Operator=OR
  Multiport Switch : MultiPortSwitch  zeroidx=off  SaturateOnIntegerOverflow=on
  NEGATIVE Edge : Subsystem  AncestorBlock=extra_sc/Edge/POSITIVE Edge  TreatAsAtomicUnit=on
  POSITIVE Edge : Subsystem  AncestorBlock=extra_sc/Delay_discrete/OFF Delay  TreatAsAtomicUnit=on
  Unit Delay : UnitDelay  X0=ic  SampleTime=Ts
  either edge : Constant  Value=[1 1]
  neg. edge : Constant  Value=[0 1]
  pos. edge : Constant  Value=[1 0]
  Out : Outport
  wires:
  either edge/1 -> Multiport Switch/4
  Demux/2 -> NEGATIVE Edge/Enable
  Demux/1 -> POSITIVE Edge/Enable
  Multiport Switch/1 -> Demux/1
  Constant1/1 -> Multiport Switch/1
  neg. edge/1 -> Multiport Switch/3
  pos. edge/1 -> Multiport Switch/2
  In/1 -> Unit Delay/1, NEGATIVE Edge/1(IN), POSITIVE Edge/1(IN)
  Unit Delay/1 -> NEGATIVE Edge/2(IN previous), POSITIVE Edge/2(IN previous)
  POSITIVE Edge/1(OUT) -> Logical Operator1/1
  NEGATIVE Edge/1(OUT) -> Logical Operator1/2
  Logical Operator1/1 -> Out/1

== system CSWI/CSWI/Блок включения/ClsTmms3/OFF Delay ==
  IN : Inport
  DELAY : Inport  Port=2
  Enable : EnablePort  PropagateVarSize=During execution
  Constant2 : Constant  Value=-Ts
  Constant3 : Constant  Value=Ts
  Discrete Edge Detector : powerlib_extras/Discrete  Control Blocks/Discrete Edge Detector  model=Falling  ic=ic  Ts=Ts
  Logical Operator1 : Logic
  Logical Operator2 : Logic  Operator=NOT
  Logical Operator3 : Logic  Operator=NOT
  Relational Operator : RelationalOperator  OutDataTypeStr=boolean  InputSameDT=on
  Sum1 : Sum  Inputs=+-  SaturateOnIntegerOverflow=on  InputSameDT=on  OutDataTypeStr=Inherit: Same as first input
  Switch : Switch  Threshold=0.5  SaturateOnIntegerOverflow=on  InputSameDT=on
  Unit Delay : UnitDelay  SampleTime=Ts
  OUT : Outport
  wires:
  Unit Delay/1 -> Switch/3
  Sum1/1 -> Relational Operator/2, Unit Delay/1
  Switch/1 -> Sum1/1
  Constant3/1 -> Sum1/2
  Relational Operator/1 -> Logical Operator1/2
  IN/1 -> Discrete Edge Detector/1, Logical Operator2/1
  Logical Operator1/1 -> Logical Operator3/1
  DELAY/1 -> Switch/1
  Discrete Edge Detector/1 -> Switch/2
  Constant2/1 -> Relational Operator/1
  Logical Operator2/1 -> Logical Operator1/1
  Logical Operator3/1 -> OUT/1

== system CSWI/CSWI/Блок включения/ClsTmms3/ON Delay ==
  IN : Inport
  DELAY : Inport  Port=2
  Enable : EnablePort  PropagateVarSize=During execution
  Constant2 : Constant  Value=-Ts
  Constant3 : Constant  Value=Ts
  Discrete Edge Detector : powerlib_extras/Discrete  Control Blocks/Discrete Edge Detector  model=Rising  ic=ic  Ts=Ts
  Logical Operator1 : Logic
  Relational Operator : RelationalOperator  OutDataTypeStr=boolean  InputSameDT=on
  Sum1 : Sum  Inputs=+-  SaturateOnIntegerOverflow=on  InputSameDT=on  OutDataTypeStr=Inherit: Same as first input
  Switch : Switch  Threshold=0.5  SaturateOnIntegerOverflow=on  InputSameDT=on
  Unit Delay : UnitDelay  SampleTime=Ts
  OUT : Outport
  wires:
  Unit Delay/1 -> Switch/3
  Sum1/1 -> Unit Delay/1, Relational Operator/2
  Switch/1 -> Sum1/1
  Constant3/1 -> Sum1/2
  Relational Operator/1 -> Logical Operator1/2
  IN/1 -> Discrete Edge Detector/1, Logical Operator1/1
  Logical Operator1/1 -> OUT/1
  DELAY/1 -> Switch/1
  Discrete Edge Detector/1 -> Switch/2
  Constant2/1 -> Relational Operator/1

== system CSWI/CSWI/Блок включения/ClsTmms4/OFF Delay ==
  IN : Inport
  DELAY : Inport  Port=2
  Enable : EnablePort  PropagateVarSize=During execution
  Constant2 : Constant  Value=-Ts
  Constant3 : Constant  Value=Ts
  Discrete Edge Detector : powerlib_extras/Discrete  Control Blocks/Discrete Edge Detector  model=Falling  ic=ic  Ts=Ts
  Logical Operator1 : Logic
  Logical Operator2 : Logic  Operator=NOT
  Logical Operator3 : Logic  Operator=NOT
  Relational Operator : RelationalOperator  OutDataTypeStr=boolean  InputSameDT=on
  Sum1 : Sum  Inputs=+-  SaturateOnIntegerOverflow=on  InputSameDT=on  OutDataTypeStr=Inherit: Same as first input
  Switch : Switch  Threshold=0.5  SaturateOnIntegerOverflow=on  InputSameDT=on
  Unit Delay : UnitDelay  SampleTime=Ts
  OUT : Outport
  wires:
  Unit Delay/1 -> Switch/3
  Sum1/1 -> Relational Operator/2, Unit Delay/1
  Switch/1 -> Sum1/1
  Constant3/1 -> Sum1/2
  Relational Operator/1 -> Logical Operator1/2
  IN/1 -> Discrete Edge Detector/1, Logical Operator2/1
  Logical Operator1/1 -> Logical Operator3/1
  DELAY/1 -> Switch/1
  Discrete Edge Detector/1 -> Switch/2
  Constant2/1 -> Relational Operator/1
  Logical Operator2/1 -> Logical Operator1/1
  Logical Operator3/1 -> OUT/1

== system CSWI/CSWI/Блок включения/ClsTmms4/ON Delay ==
  IN : Inport
  DELAY : Inport  Port=2
  Enable : EnablePort  PropagateVarSize=During execution
  Constant2 : Constant  Value=-Ts
  Constant3 : Constant  Value=Ts
  Discrete Edge Detector : powerlib_extras/Discrete  Control Blocks/Discrete Edge Detector  model=Rising  ic=ic  Ts=Ts
  Logical Operator1 : Logic
  Relational Operator : RelationalOperator  OutDataTypeStr=boolean  InputSameDT=on
  Sum1 : Sum  Inputs=+-  SaturateOnIntegerOverflow=on  InputSameDT=on  OutDataTypeStr=Inherit: Same as first input
  Switch : Switch  Threshold=0.5  SaturateOnIntegerOverflow=on  InputSameDT=on
  Unit Delay : UnitDelay  SampleTime=Ts
  OUT : Outport
  wires:
  Unit Delay/1 -> Switch/3
  Sum1/1 -> Unit Delay/1, Relational Operator/2
  Switch/1 -> Sum1/1
  Constant3/1 -> Sum1/2
  Relational Operator/1 -> Logical Operator1/2
  IN/1 -> Discrete Edge Detector/1, Logical Operator1/1
  Logical Operator1/1 -> OUT/1
  DELAY/1 -> Switch/1
  Discrete Edge Detector/1 -> Switch/2
  Constant2/1 -> Relational Operator/1

== system CSWI/CSWI/Блок включения/Discrete Bistable7/RESET Priority ==
  S : Inport
  R : Inport  Port=2
  Enable : EnablePort  PropagateVarSize=During execution
  IC = ic : UnitDelay  X0=ic  SampleTime=Ts
  Logical Operator : Logic  Operator=OR
  Logical Operator1 : Logic  Operator=NOT  Inputs=1
  Logical Operator2 : Logic
  Logical Operator3 : Logic  Operator=NOT  Inputs=1
  Q : Outport
  !Q : Outport  Port=2
  wires:
  Logical Operator2/1 -> Q/1, Logical Operator3/1, IC = ic/1
  Logical Operator1/1 -> Logical Operator2/2
  R/1 -> Logical Operator1/1
  Logical Operator/1 -> Logical Operator2/1
  IC = ic/1 -> Logical Operator/2
  Logical Operator3/1 -> !Q/1
  S/1 -> Logical Operator/1

== system CSWI/CSWI/Блок включения/Discrete Bistable7/SET  Priority ==
  S : Inport
  R : Inport  Port=2
  Enable : EnablePort  PropagateVarSize=During execution
  IC = ic : UnitDelay  X0=ic  SampleTime=Ts
  Logical Operator : Logic  Operator=OR
  Logical Operator1 : Logic  Operator=NOT  Inputs=1
  Logical Operator2 : Logic
  Logical Operator3 : Logic  Operator=NOT  Inputs=1
  Q : Outport
  !Q : Outport  Port=2
  wires:
  S/1 -> Logical Operator/1
  Logical Operator3/1 -> !Q/1
  Logical Operator/1 -> IC = ic/1, Logical Operator3/1, Q/1
  R/1 -> Logical Operator1/1
  Logical Operator1/1 -> Logical Operator2/1
  IC = ic/1 -> Logical Operator2/2
  Logical Operator2/1 -> Logical Operator/2

== system CSWI/CSWI/Блок отключения/OpnTmms1/OFF Delay ==
  IN : Inport
  DELAY : Inport  Port=2
  Enable : EnablePort  PropagateVarSize=During execution
  Constant2 : Constant  Value=-Ts
  Constant3 : Constant  Value=Ts
  Discrete Edge Detector : powerlib_extras/Discrete  Control Blocks/Discrete Edge Detector  model=Falling  ic=ic  Ts=Ts
  Logical Operator1 : Logic
  Logical Operator2 : Logic  Operator=NOT
  Logical Operator3 : Logic  Operator=NOT
  Relational Operator : RelationalOperator  OutDataTypeStr=boolean  InputSameDT=on
  Sum1 : Sum  Inputs=+-  SaturateOnIntegerOverflow=on  InputSameDT=on  OutDataTypeStr=Inherit: Same as first input
  Switch : Switch  Threshold=0.5  SaturateOnIntegerOverflow=on  InputSameDT=on
  Unit Delay : UnitDelay  SampleTime=Ts
  OUT : Outport
  wires:
  Unit Delay/1 -> Switch/3
  Sum1/1 -> Relational Operator/2, Unit Delay/1
  Switch/1 -> Sum1/1
  Constant3/1 -> Sum1/2
  Relational Operator/1 -> Logical Operator1/2
  IN/1 -> Discrete Edge Detector/1, Logical Operator2/1
  Logical Operator1/1 -> Logical Operator3/1
  DELAY/1 -> Switch/1
  Discrete Edge Detector/1 -> Switch/2
  Constant2/1 -> Relational Operator/1
  Logical Operator2/1 -> Logical Operator1/1
  Logical Operator3/1 -> OUT/1

== system CSWI/CSWI/Блок отключения/OpnTmms1/ON Delay ==
  IN : Inport
  DELAY : Inport  Port=2
  Enable : EnablePort  PropagateVarSize=During execution
  Constant2 : Constant  Value=-Ts
  Constant3 : Constant  Value=Ts
  Discrete Edge Detector : powerlib_extras/Discrete  Control Blocks/Discrete Edge Detector  model=Rising  ic=ic  Ts=Ts
  Logical Operator1 : Logic
  Relational Operator : RelationalOperator  OutDataTypeStr=boolean  InputSameDT=on
  Sum1 : Sum  Inputs=+-  SaturateOnIntegerOverflow=on  InputSameDT=on  OutDataTypeStr=Inherit: Same as first input
  Switch : Switch  Threshold=0.5  SaturateOnIntegerOverflow=on  InputSameDT=on
  Unit Delay : UnitDelay  SampleTime=Ts
  OUT : Outport
  wires:
  Unit Delay/1 -> Switch/3
  Sum1/1 -> Unit Delay/1, Relational Operator/2
  Switch/1 -> Sum1/1
  Constant3/1 -> Sum1/2
  Relational Operator/1 -> Logical Operator1/2
  IN/1 -> Discrete Edge Detector/1, Logical Operator1/1
  Logical Operator1/1 -> OUT/1
  DELAY/1 -> Switch/1
  Discrete Edge Detector/1 -> Switch/2
  Constant2/1 -> Relational Operator/1

== system CSWI/CSWI/Блок отключения/OpnTmms2/Edge_Detector ==
  note: Edge or Slope Detector
  note: Silvano Casoria
      | Power System Simulation Laboratory
      | IREQ, Hydro-Quebc
  In : Inport
  Constant1 : Constant  Value=model
  Demux : Demux  Outputs=2
  Logical Operator1 : Logic  Operator=OR
  Multiport Switch : MultiPortSwitch  zeroidx=off  SaturateOnIntegerOverflow=on
  NEGATIVE Edge : Subsystem  AncestorBlock=extra_sc/Edge/POSITIVE Edge  TreatAsAtomicUnit=on
  POSITIVE Edge : Subsystem  AncestorBlock=extra_sc/Delay_discrete/OFF Delay  TreatAsAtomicUnit=on
  Unit Delay : UnitDelay  X0=ic  SampleTime=Ts
  either edge : Constant  Value=[1 1]
  neg. edge : Constant  Value=[0 1]
  pos. edge : Constant  Value=[1 0]
  Out : Outport
  wires:
  either edge/1 -> Multiport Switch/4
  Demux/2 -> NEGATIVE Edge/Enable
  Demux/1 -> POSITIVE Edge/Enable
  Multiport Switch/1 -> Demux/1
  Constant1/1 -> Multiport Switch/1
  neg. edge/1 -> Multiport Switch/3
  pos. edge/1 -> Multiport Switch/2
  In/1 -> Unit Delay/1, NEGATIVE Edge/1(IN), POSITIVE Edge/1(IN)
  Unit Delay/1 -> NEGATIVE Edge/2(IN previous), POSITIVE Edge/2(IN previous)
  POSITIVE Edge/1(OUT) -> Logical Operator1/1
  NEGATIVE Edge/1(OUT) -> Logical Operator1/2
  Logical Operator1/1 -> Out/1

== system CSWI/CSWI/Блок отключения/OpnTmms3/OFF Delay ==
  IN : Inport
  DELAY : Inport  Port=2
  Enable : EnablePort  PropagateVarSize=During execution
  Constant2 : Constant  Value=-Ts
  Constant3 : Constant  Value=Ts
  Discrete Edge Detector : powerlib_extras/Discrete  Control Blocks/Discrete Edge Detector  model=Falling  ic=ic  Ts=Ts
  Logical Operator1 : Logic
  Logical Operator2 : Logic  Operator=NOT
  Logical Operator3 : Logic  Operator=NOT
  Relational Operator : RelationalOperator  OutDataTypeStr=boolean  InputSameDT=on
  Sum1 : Sum  Inputs=+-  SaturateOnIntegerOverflow=on  InputSameDT=on  OutDataTypeStr=Inherit: Same as first input
  Switch : Switch  Threshold=0.5  SaturateOnIntegerOverflow=on  InputSameDT=on
  Unit Delay : UnitDelay  SampleTime=Ts
  OUT : Outport
  wires:
  Unit Delay/1 -> Switch/3
  Sum1/1 -> Relational Operator/2, Unit Delay/1
  Switch/1 -> Sum1/1
  Constant3/1 -> Sum1/2
  Relational Operator/1 -> Logical Operator1/2
  IN/1 -> Discrete Edge Detector/1, Logical Operator2/1
  Logical Operator1/1 -> Logical Operator3/1
  DELAY/1 -> Switch/1
  Discrete Edge Detector/1 -> Switch/2
  Constant2/1 -> Relational Operator/1
  Logical Operator2/1 -> Logical Operator1/1
  Logical Operator3/1 -> OUT/1

== system CSWI/CSWI/Блок отключения/OpnTmms3/ON Delay ==
  IN : Inport
  DELAY : Inport  Port=2
  Enable : EnablePort  PropagateVarSize=During execution
  Constant2 : Constant  Value=-Ts
  Constant3 : Constant  Value=Ts
  Discrete Edge Detector : powerlib_extras/Discrete  Control Blocks/Discrete Edge Detector  model=Rising  ic=ic  Ts=Ts
  Logical Operator1 : Logic
  Relational Operator : RelationalOperator  OutDataTypeStr=boolean  InputSameDT=on
  Sum1 : Sum  Inputs=+-  SaturateOnIntegerOverflow=on  InputSameDT=on  OutDataTypeStr=Inherit: Same as first input
  Switch : Switch  Threshold=0.5  SaturateOnIntegerOverflow=on  InputSameDT=on
  Unit Delay : UnitDelay  SampleTime=Ts
  OUT : Outport
  wires:
  Unit Delay/1 -> Switch/3
  Sum1/1 -> Unit Delay/1, Relational Operator/2
  Switch/1 -> Sum1/1
  Constant3/1 -> Sum1/2
  Relational Operator/1 -> Logical Operator1/2
  IN/1 -> Discrete Edge Detector/1, Logical Operator1/1
  Logical Operator1/1 -> OUT/1
  DELAY/1 -> Switch/1
  Discrete Edge Detector/1 -> Switch/2
  Constant2/1 -> Relational Operator/1

== system CSWI/CSWI/Положение блок-контактов/BlkTmms1/OFF Delay ==
  IN : Inport
  DELAY : Inport  Port=2
  Enable : EnablePort  PropagateVarSize=During execution
  Constant2 : Constant  Value=-Ts
  Constant3 : Constant  Value=Ts
  Discrete Edge Detector : powerlib_extras/Discrete  Control Blocks/Discrete Edge Detector  model=Falling  ic=ic  Ts=Ts
  Logical Operator1 : Logic
  Logical Operator2 : Logic  Operator=NOT
  Logical Operator3 : Logic  Operator=NOT
  Relational Operator : RelationalOperator  OutDataTypeStr=boolean  InputSameDT=on
  Sum1 : Sum  Inputs=+-  SaturateOnIntegerOverflow=on  InputSameDT=on  OutDataTypeStr=Inherit: Same as first input
  Switch : Switch  Threshold=0.5  SaturateOnIntegerOverflow=on  InputSameDT=on
  Unit Delay : UnitDelay  SampleTime=Ts
  OUT : Outport
  wires:
  Unit Delay/1 -> Switch/3
  Sum1/1 -> Relational Operator/2, Unit Delay/1
  Switch/1 -> Sum1/1
  Constant3/1 -> Sum1/2
  Relational Operator/1 -> Logical Operator1/2
  IN/1 -> Discrete Edge Detector/1, Logical Operator2/1
  Logical Operator1/1 -> Logical Operator3/1
  DELAY/1 -> Switch/1
  Discrete Edge Detector/1 -> Switch/2
  Constant2/1 -> Relational Operator/1
  Logical Operator2/1 -> Logical Operator1/1
  Logical Operator3/1 -> OUT/1
